simulink library "singleTether_cl"  (R2018b)
settings: Solver=VariableStepAuto  StartTime=0.0  StopTime=10.0  RelTol=1e-3
values from neighbouring files (symbols this model uses):
  ini_Ri_o = Ri_o    [singleTether_ts.m]
  ini_Vi_o = zeros(size(Vi_o))    [singleTether_ts.m]
  initNodePoss = [linspace(ini_R1_o(1),ini_Rn_o(1),N);     linspace(ini_R1_o(2),ini_Rn_o(2),N);     linspace(ini_R1_o(3),ini_Rn_o(3),N)]    [singleTether_init.m]
  initNodeVels = zeros(size(initNodePoss))    [singleTether_init.m]
undefined symbols (not defined in the file or in its folder): gnd_station, ini_euler_ang, ini_Rcm_o, R11_g, R1n_cm, rotation_sequence, sim_param
libraries: tetherBuoyancyAndWeight_ul x1, tetherDragForce_ul x1, tetherInternalForces_ul x1
settings Model: Creator=asiddiq2  LastModifiedBy=asiddiq2

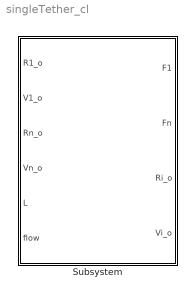
== system singleTether_cl ==
  Subsystem : Subsystem  mask{N=sim_param.N, dia_t=sim_param.tether_param.tether_diameter(1), E=sim_param.tether_param.tether_youngs, rho_tether=sim_param.tether_param.tether_density+ sim_param.env_param.density, Cd=sim_param.tether_param.CD_cylinder, zeta=sim_param.tether_param.damping_ratio, rho=sim_param.env_param.density, g=sim_param.env_param.grav, mass=sim_param.geom_param.mass, ini_Rn_o=ini_Rcm_o + rotation_sequence(ini_euler_ang)*R1n_cm, ini_R1_o=gnd_station + R11_g}
      mask prompts: N "Number of nodes (N>=2)"; dia_t "Tether diameter (m)"; E "Tether youngs modulus (N/m^2)"; rho_tether "Tether density (kg/m^3)"; Cd "Tether drag coefficient"; zeta "Damping ratio"; rho "Fluid density"; g "Gravitational acceleration"; mass "Vehicle mass"; ini_Rn_o "Initial vehicle attachment position vector"; ini_R1_o "Initial ground attachment position vector"
      mask init:
      | singleTether_init
      mask DialogControl Container2 Prompt: Tether properties

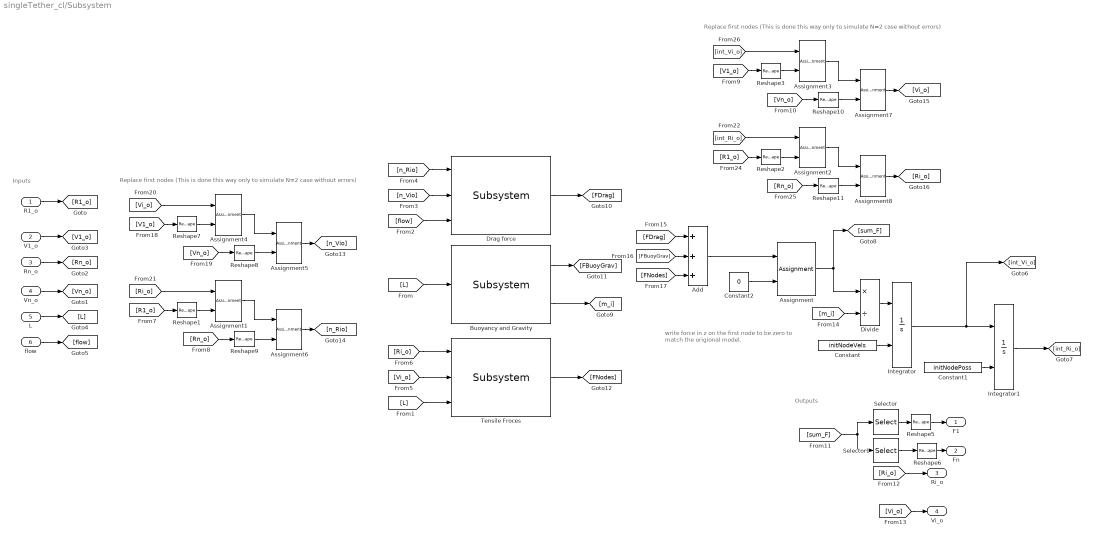
== system singleTether_cl/Subsystem ==
  note: write force in z on the first node to be zero
      | to match the origional model.
  note: Replace first nodes (This is done this way only to simulate N=2 case
      | without errors)
  note: Outputs
  note: Inputs
  note: Replace first nodes (This is done this way only to simulate N=2 case
      | without errors)
  R1_o : Inport
  V1_o : Inport  Port=2
  Rn_o : Inport  Port=3
  Vn_o : Inport  Port=4
  L : Inport  Port=5
  flow : Inport  Port=6
  Add : Sum  Inputs=+++
  Assignment : Assignment  NumberOfDimensions=2  DiagnosticForDimensions=Warning  IndexOptions=Index vector (dialog),Index vector (dialog)  Indices=3,1  OutputSizes=1,1
  Assignment{1..4} (4 alike) : Assignment  NumberOfDimensions=2  DiagnosticForDimensions=Warning  IndexOptions=Assign all,Index vector (dialog)  Indices=1,1  OutputSizes=1,1
  Assignment{5..8} (4 alike) : Assignment  NumberOfDimensions=2  DiagnosticForDimensions=Warning  IndexOptions=Assign all,Index vector (dialog)  Indices=1,N  OutputSizes=1,1
  Buoyancy and Gravity : tetherBuoyancyAndWeight_ul/Subsystem  N=N  dia_t=dia_t  rho_fluid=rho  rho_tether=rho_tether  g=g
  Constant : Constant  Value=initNodeVels
  Constant1 : Constant  Value=initNodePoss
  Constant2 : Constant  Value=0
  Divide : Product  Inputs=*/
  Drag force : tetherDragForce_ul/Subsystem  Cd=Cd  rho_fluid=rho  dia_t=dia_t
  Integrator : Integrator  InitialConditionSource=external  InitialCondition=ini_Vi_o
  Integrator1 : Integrator  InitialConditionSource=external  InitialCondition=ini_Ri_o
  Reshape{1..3,5..11} (10 alike) : Reshape  OutputDimensionality=Column vector (2-D)
  Selector : Selector  NumberOfDimensions=2  InputPortWidth=3  IndexOptions=Select all,Index vector (dialog)  Indices=[1],1  OutputSizes=1,1
  Selector1 : Selector  NumberOfDimensions=2  InputPortWidth=3  IndexOptions=Select all,Index vector (dialog)  Indices=[N],N  OutputSizes=1,1
  Tensile Froces : tetherInternalForces_ul/Subsystem  N=N  E=E  dia_t=dia_t  mass=mass  zeta=zeta
  F1 : Outport
  Fn : Outport  Port=2
  Ri_o : Outport  Port=3
  Vi_o : Outport  Port=4
  wires:
  R1_o/1 -> [R1_o]
  V1_o/1 -> [V1_o]
  Rn_o/1 -> [Rn_o]
  Vn_o/1 -> [Vn_o]
  L/1 -> [L]
  flow/1 -> [flow]
  [L] -> Buoyancy and Gravity/1
  [L] -> Tensile Froces/3
  [flow] -> Drag force/3
  Buoyancy and Gravity/1 -> [FBuoyGrav]
  Drag force/1 -> [FDrag]
  Tensile Froces/1 -> [FNodes]
  Divide/1 -> Integrator/1
  [n_Rio] -> Drag force/1
  [Vi_o] -> Tensile Froces/2
  [Ri_o] -> Tensile Froces/1
  Integrator/1 -> [int_Vi_o], Integrator1/1
  [sum_F] -> Selector/1, Selector1/1
  [Ri_o] -> Ri_o/1
  [Vi_o] -> Vi_o/1
  Selector1/1 -> Reshape6/1
  Reshape6/1 -> Fn/1
  Selector/1 -> Reshape5/1
  Reshape5/1 -> F1/1
  Constant/1 -> Integrator/2
  Constant1/1 -> Integrator1/2
  Buoyancy and Gravity/2 -> [m_i]
  [m_i] -> Divide/2
  [FBuoyGrav] -> Add/2
  [FDrag] -> Add/1
  [FNodes] -> Add/3
  Reshape7/1 -> Assignment4/2
  [V1_o] -> Reshape7/1
  [Vi_o] -> Assignment4/1
  [Vn_o] -> Reshape8/1
  Reshape8/1 -> Assignment5/2
  Assignment4/1 -> Assignment5/1
  Assignment5/1 -> [n_Vio]
  [n_Vio] -> Drag force/2
  Assignment1/1 -> Assignment6/1
  [R1_o] -> Reshape1/1
  [Rn_o] -> Reshape9/1
  Assignment6/1 -> [n_Rio]
  [Ri_o] -> Assignment1/1
  Reshape1/1 -> Assignment1/2
  Reshape9/1 -> Assignment6/2
  Integrator1/1 -> [int_Ri_o]
  [V1_o] -> Reshape3/1
  Reshape3/1 -> Assignment3/2
  Assignment3/1 -> Assignment7/1
  Reshape11/1 -> Assignment8/2
  [int_Vi_o] -> Assignment3/1
  [R1_o] -> Reshape2/1
  [Vn_o] -> Reshape10/1
  [Rn_o] -> Reshape11/1
  Assignment7/1 -> [Vi_o]
  Assignment2/1 -> Assignment8/1
  [int_Ri_o] -> Assignment2/1
  Reshape10/1 -> Assignment7/2
  Assignment8/1 -> [Ri_o]
  Reshape2/1 -> Assignment2/2
  Assignment/1 -> [sum_F], Divide/1
  Add/1 -> Assignment/1
  Constant2/1 -> Assignment/2
